simulink model "TesteEloGhendy"  (R2021b)
settings: Solver=FixedStepAuto  StartTime=0.0  StopTime=TempoSimulacao  RelTol=1e-3
values from neighbouring files (symbols this model uses):
  FatorSimulacao = 1e-3    (= 0.001)    [TesteRealCurtoFuses.m]    (also in TesteRealCurto_SemFuse.m)
  le = 1e-10    [TesteRealCurto.m]    (also in TesteRealCurtoFuses.m; TesteRealCurto_SemFuse.m)
  lm = (imag(Zm)/(2*pi*f))*d    [TesteRealCurto.m]    (also in TesteRealCurtoFuses.m; TesteRealCurto_SemFuse.m)
  lp = (imag(Zp)/(2*pi*f))*d    [TesteRealCurto.m]    (also in TesteRealCurtoFuses.m; TesteRealCurto_SemFuse.m)
  NRE = 1e-12    [TesteRealCurto.m]    (also in TesteRealCurtoFuses.m; TesteRealCurto_SemFuse.m)
  rm = real(Zm)*d    [TesteRealCurto.m]    (also in TesteRealCurtoFuses.m; TesteRealCurto_SemFuse.m)
  rp = real(Zp)*d    [TesteRealCurto.m]    (also in TesteRealCurtoFuses.m; TesteRealCurto_SemFuse.m)
  rtc = 10    [TesteRealCurto.m]    (also in TesteRealCurtoFuses.m; TesteRealCurto_SemFuse.m)
  rti = 10    [TesteRealCurto.m]    (also in TesteRealCurtoFuses.m; TesteRealCurto_SemFuse.m)
undefined symbols (not defined in the file or in its folder): D11, Delta, POT, PotConsumidor, Ra_Curto, Rb_Curto, Rc_Curto
libraries: spsRMSLib x15, spsBreakerLib x7, spsCurrentMeasurementLib x7, spsSeriesRLCBranchLib x6, spsThreePhaseVIMeasurementLib x4, spsThreePhaseTransformerTwoWindingsLib x2, spsThreePhaseSeriesRLCLoadLib x1, spsThreePhaseBreakerLib x1, spsThreePhaseSourceLib x1, spsMutualInductanceLib x1, spspowerguiLib x1
(part 2 of 2)

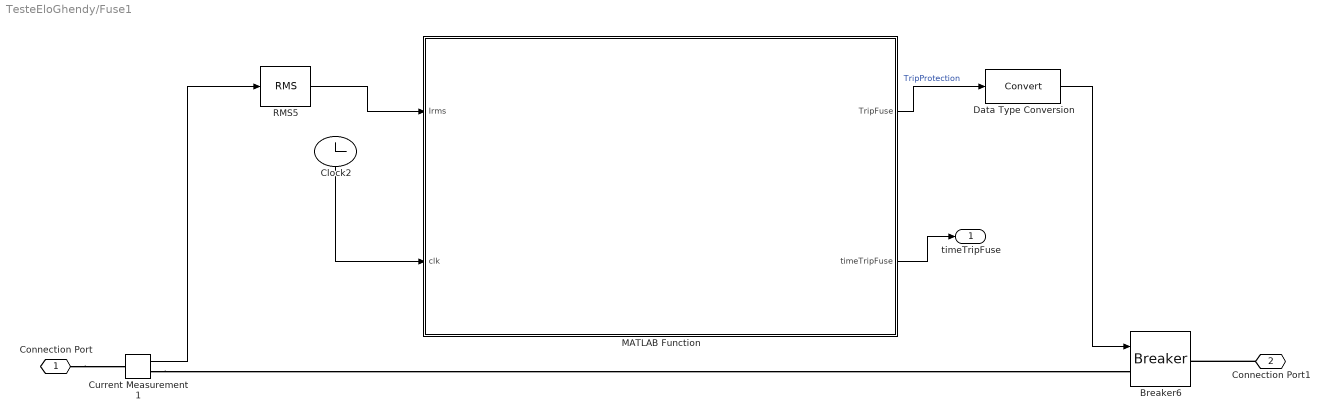
== system TesteEloGhendy/Fuse1 ==
  Breaker6 : spsBreakerLib/Breaker  InitialState=1  SwitchingTimes="[1/60  5/60]"  External=on  BreakerResistance=0.01  SnubberResistance=1e6  SnubberCapacitance=inf  Measurements=None  MoreParameters=on  NoBreakLoop=off
      settings: SourceProductBaseCode=PS
  Clock2 : Clock
      settings: Decimation=1000
  Current Measurement1 : spsCurrentMeasurementLib/Current Measurement  PhasorSimulation=off  OutputType=Complex  PSBequivalent=0
  Data Type Conversion : DataTypeConversion
  MATLAB Function : MATLAB Function
  RMS5 : spsRMSLib/RMS  TrueRMS=on  Freq=60  RMSInit=0  Ts=0
  Connection Port : PMIOPort  Side=Right
  Connection Port1 : PMIOPort  Port=2  Side=Left
  timeTripFuse : Outport
  wires:
  MATLAB Function/1(TripFuse) -> Data Type Conversion/1  "TripProtection"
  RMS5/1 -> MATLAB Function/1(Irms)
  Data Type Conversion/1 -> Breaker6/1
  Current Measurement1/1 -> RMS5/1
  Clock2/1 -> MATLAB Function/2(clk)
  MATLAB Function/2(timeTripFuse) -> timeTripFuse/1
  connections:
  Current Measurement1/RConn1 -- Breaker6/LConn1
  Connection Port/RConn1 -- Current Measurement1/LConn1
  Connection Port1/RConn1 -- Breaker6/RConn1

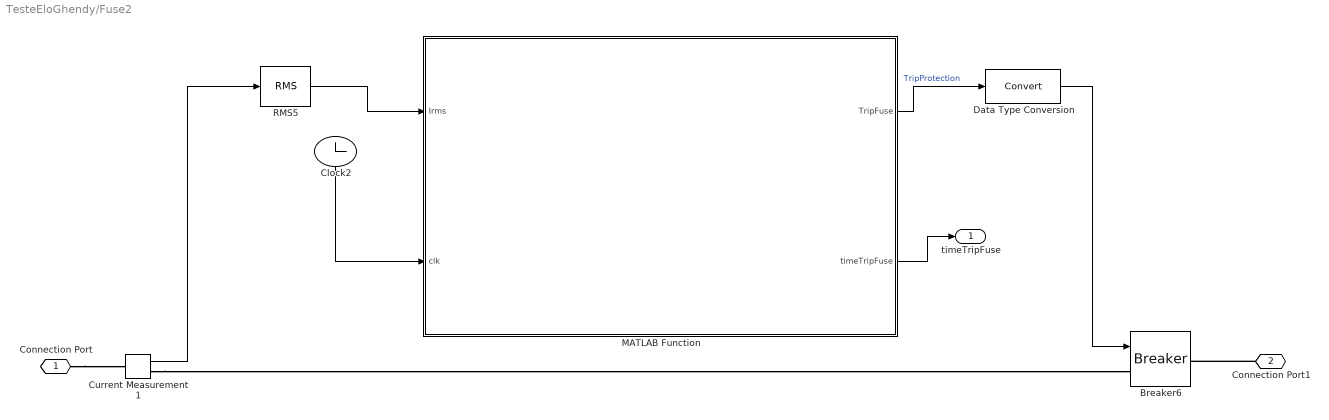
== system TesteEloGhendy/Fuse2 ==
  Breaker6 : spsBreakerLib/Breaker  InitialState=1  SwitchingTimes="[1/60  5/60]"  External=on  BreakerResistance=0.01  SnubberResistance=1e6  SnubberCapacitance=inf  Measurements=None  MoreParameters=on  NoBreakLoop=off
      settings: SourceProductBaseCode=PS
  Clock2 : Clock
      settings: Decimation=1000
  Current Measurement1 : spsCurrentMeasurementLib/Current Measurement  PhasorSimulation=off  OutputType=Complex  PSBequivalent=0
  Data Type Conversion : DataTypeConversion
  MATLAB Function : MATLAB Function
  RMS5 : spsRMSLib/RMS  TrueRMS=on  Freq=60  RMSInit=0  Ts=0
  Connection Port : PMIOPort  Side=Right
  Connection Port1 : PMIOPort  Port=2  Side=Left
  timeTripFuse : Outport
  wires:
  MATLAB Function/1(TripFuse) -> Data Type Conversion/1  "TripProtection"
  RMS5/1 -> MATLAB Function/1(Irms)
  Data Type Conversion/1 -> Breaker6/1
  Current Measurement1/1 -> RMS5/1
  Clock2/1 -> MATLAB Function/2(clk)
  MATLAB Function/2(timeTripFuse) -> timeTripFuse/1
  connections:
  Current Measurement1/RConn1 -- Breaker6/LConn1
  Connection Port/RConn1 -- Current Measurement1/LConn1
  Connection Port1/RConn1 -- Breaker6/RConn1

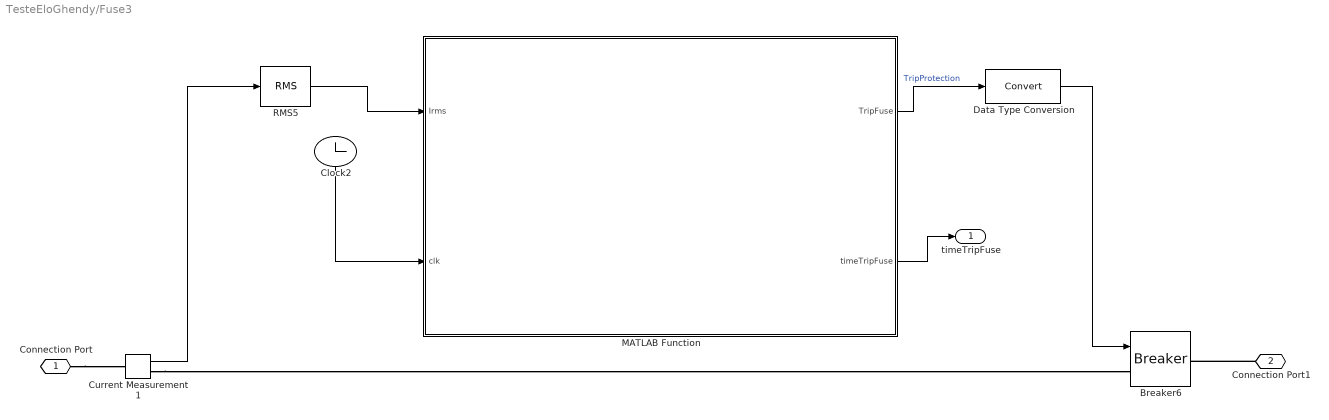
== system TesteEloGhendy/Fuse3 ==
  Breaker6 : spsBreakerLib/Breaker  InitialState=1  SwitchingTimes="[1/60  5/60]"  External=on  BreakerResistance=0.01  SnubberResistance=1e6  SnubberCapacitance=inf  Measurements=None  MoreParameters=on  NoBreakLoop=off
      settings: SourceProductBaseCode=PS
  Clock2 : Clock
      settings: Decimation=1000
  Current Measurement1 : spsCurrentMeasurementLib/Current Measurement  PhasorSimulation=off  OutputType=Complex  PSBequivalent=0
  Data Type Conversion : DataTypeConversion
  MATLAB Function : MATLAB Function
  RMS5 : spsRMSLib/RMS  TrueRMS=on  Freq=60  RMSInit=0  Ts=0
  Connection Port : PMIOPort  Side=Right
  Connection Port1 : PMIOPort  Port=2  Side=Left
  timeTripFuse : Outport
  wires:
  MATLAB Function/1(TripFuse) -> Data Type Conversion/1  "TripProtection"
  RMS5/1 -> MATLAB Function/1(Irms)
  Data Type Conversion/1 -> Breaker6/1
  Current Measurement1/1 -> RMS5/1
  Clock2/1 -> MATLAB Function/2(clk)
  MATLAB Function/2(timeTripFuse) -> timeTripFuse/1
  connections:
  Current Measurement1/RConn1 -- Breaker6/LConn1
  Connection Port/RConn1 -- Current Measurement1/LConn1
  Connection Port1/RConn1 -- Breaker6/RConn1

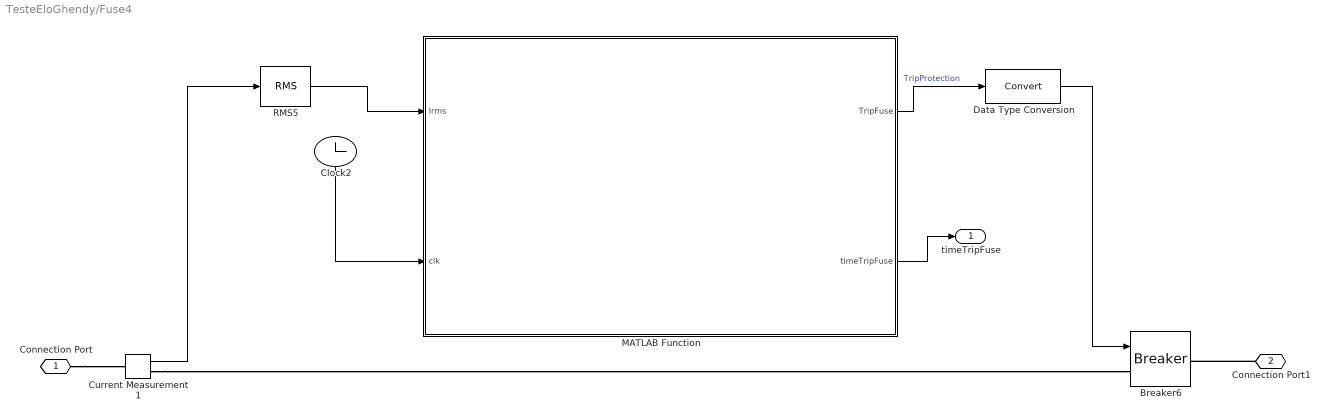
== system TesteEloGhendy/Fuse4 ==
  Breaker6 : spsBreakerLib/Breaker  InitialState=1  SwitchingTimes="[1/60  5/60]"  External=on  BreakerResistance=0.01  SnubberResistance=1e6  SnubberCapacitance=inf  Measurements=None  MoreParameters=on  NoBreakLoop=off
      settings: SourceProductBaseCode=PS
  Clock2 : Clock
      settings: Decimation=1000
  Current Measurement1 : spsCurrentMeasurementLib/Current Measurement  PhasorSimulation=off  OutputType=Complex  PSBequivalent=0
  Data Type Conversion : DataTypeConversion
  MATLAB Function : MATLAB Function
  RMS5 : spsRMSLib/RMS  TrueRMS=on  Freq=60  RMSInit=0  Ts=0
  Connection Port : PMIOPort  Side=Right
  Connection Port1 : PMIOPort  Port=2  Side=Left
  timeTripFuse : Outport
  wires:
  MATLAB Function/1(TripFuse) -> Data Type Conversion/1  "TripProtection"
  RMS5/1 -> MATLAB Function/1(Irms)
  Data Type Conversion/1 -> Breaker6/1
  Current Measurement1/1 -> RMS5/1
  Clock2/1 -> MATLAB Function/2(clk)
  MATLAB Function/2(timeTripFuse) -> timeTripFuse/1
  connections:
  Current Measurement1/RConn1 -- Breaker6/LConn1
  Connection Port/RConn1 -- Current Measurement1/LConn1
  Connection Port1/RConn1 -- Breaker6/RConn1

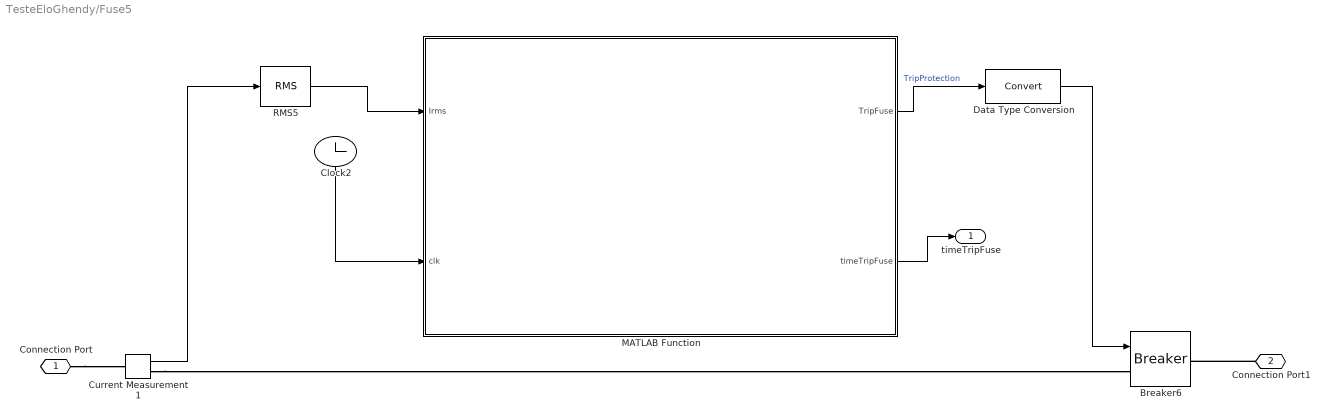
== system TesteEloGhendy/Fuse5 ==
  Breaker6 : spsBreakerLib/Breaker  InitialState=1  SwitchingTimes="[1/60  5/60]"  External=on  BreakerResistance=0.01  SnubberResistance=1e6  SnubberCapacitance=inf  Measurements=None  MoreParameters=on  NoBreakLoop=off
      settings: SourceProductBaseCode=PS
  Clock2 : Clock
      settings: Decimation=1000
  Current Measurement1 : spsCurrentMeasurementLib/Current Measurement  PhasorSimulation=off  OutputType=Complex  PSBequivalent=0
  Data Type Conversion : DataTypeConversion
  MATLAB Function : MATLAB Function
  RMS5 : spsRMSLib/RMS  TrueRMS=on  Freq=60  RMSInit=0  Ts=0
  Connection Port : PMIOPort  Side=Right
  Connection Port1 : PMIOPort  Port=2  Side=Left
  timeTripFuse : Outport
  wires:
  MATLAB Function/1(TripFuse) -> Data Type Conversion/1  "TripProtection"
  RMS5/1 -> MATLAB Function/1(Irms)
  Data Type Conversion/1 -> Breaker6/1
  Current Measurement1/1 -> RMS5/1
  Clock2/1 -> MATLAB Function/2(clk)
  MATLAB Function/2(timeTripFuse) -> timeTripFuse/1
  connections:
  Current Measurement1/RConn1 -- Breaker6/LConn1
  Connection Port/RConn1 -- Current Measurement1/LConn1
  Connection Port1/RConn1 -- Breaker6/RConn1

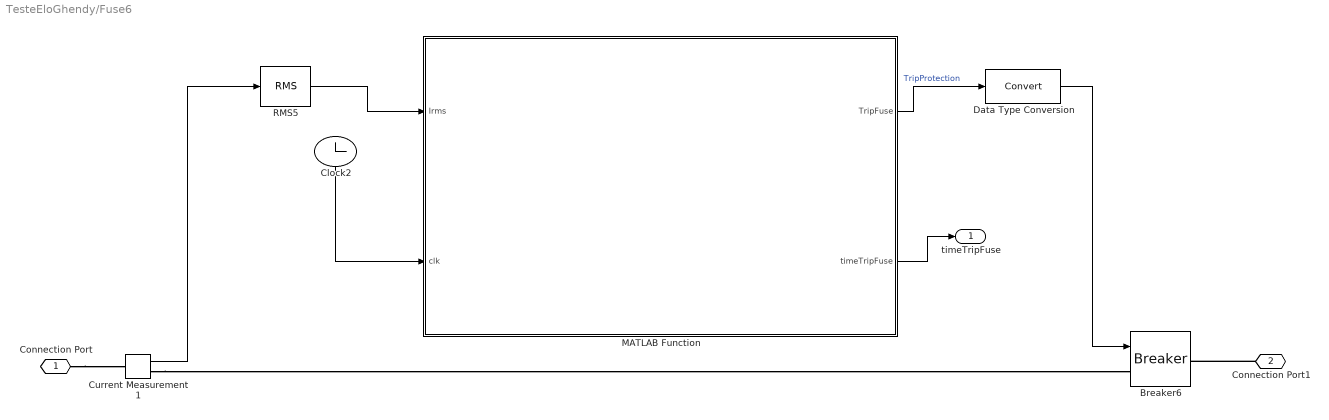
== system TesteEloGhendy/Fuse6 ==
  Breaker6 : spsBreakerLib/Breaker  InitialState=1  SwitchingTimes="[1/60  5/60]"  External=on  BreakerResistance=0.01  SnubberResistance=1e6  SnubberCapacitance=inf  Measurements=None  MoreParameters=on  NoBreakLoop=off
      settings: SourceProductBaseCode=PS
  Clock2 : Clock
      settings: Decimation=1000
  Current Measurement1 : spsCurrentMeasurementLib/Current Measurement  PhasorSimulation=off  OutputType=Complex  PSBequivalent=0
  Data Type Conversion : DataTypeConversion
  MATLAB Function : MATLAB Function
  RMS5 : spsRMSLib/RMS  TrueRMS=on  Freq=60  RMSInit=0  Ts=0
  Connection Port : PMIOPort  Side=Right
  Connection Port1 : PMIOPort  Port=2  Side=Left
  timeTripFuse : Outport
  wires:
  MATLAB Function/1(TripFuse) -> Data Type Conversion/1  "TripProtection"
  RMS5/1 -> MATLAB Function/1(Irms)
  Data Type Conversion/1 -> Breaker6/1
  Current Measurement1/1 -> RMS5/1
  Clock2/1 -> MATLAB Function/2(clk)
  MATLAB Function/2(timeTripFuse) -> timeTripFuse/1
  connections:
  Current Measurement1/RConn1 -- Breaker6/LConn1
  Connection Port/RConn1 -- Current Measurement1/LConn1
  Connection Port1/RConn1 -- Breaker6/RConn1

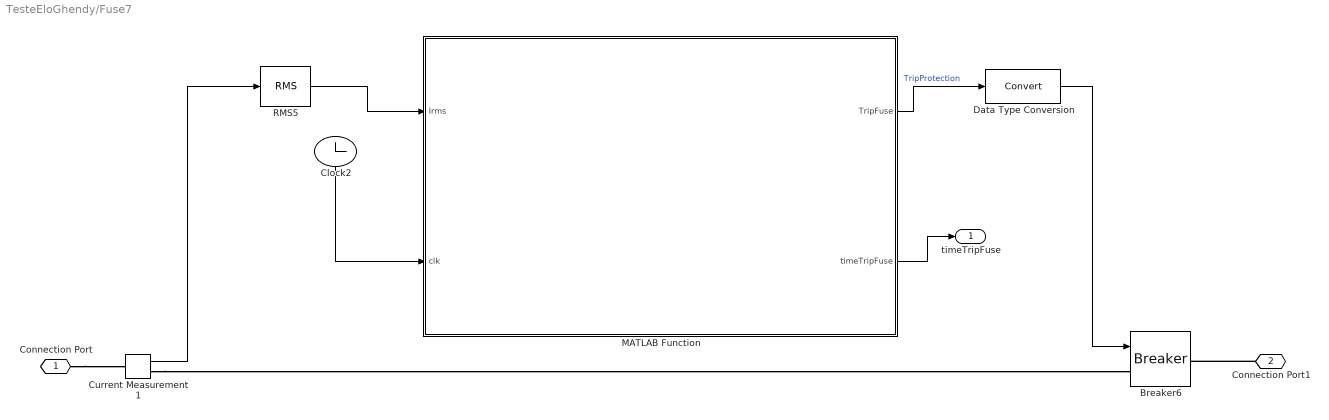
== system TesteEloGhendy/Fuse7 ==
  Breaker6 : spsBreakerLib/Breaker  InitialState=1  SwitchingTimes="[1/60  5/60]"  External=on  BreakerResistance=0.01  SnubberResistance=1e6  SnubberCapacitance=inf  Measurements=None  MoreParameters=on  NoBreakLoop=off
      settings: SourceProductBaseCode=PS
  Clock2 : Clock
      settings: Decimation=1000
  Current Measurement1 : spsCurrentMeasurementLib/Current Measurement  PhasorSimulation=off  OutputType=Complex  PSBequivalent=0
  Data Type Conversion : DataTypeConversion
  MATLAB Function : MATLAB Function
  RMS5 : spsRMSLib/RMS  TrueRMS=on  Freq=60  RMSInit=0  Ts=0
  Connection Port : PMIOPort  Side=Right
  Connection Port1 : PMIOPort  Port=2  Side=Left
  timeTripFuse : Outport
  wires:
  MATLAB Function/1(TripFuse) -> Data Type Conversion/1  "TripProtection"
  RMS5/1 -> MATLAB Function/1(Irms)
  Data Type Conversion/1 -> Breaker6/1
  Current Measurement1/1 -> RMS5/1
  Clock2/1 -> MATLAB Function/2(clk)
  MATLAB Function/2(timeTripFuse) -> timeTripFuse/1
  connections:
  Current Measurement1/RConn1 -- Breaker6/LConn1
  Connection Port/RConn1 -- Current Measurement1/LConn1
  Connection Port1/RConn1 -- Breaker6/RConn1

== matlab function TesteEloGhendy/Fuse6/MATLAB Function ==
  settings: updateMethod=DISCRETE
  data: Irms input; clk input; TripFuse output; a parameter; b parameter; c parameter; d parameter; e parameter; timeTripFuse output; IoTot parameter
function [TripFuse, timeTripFuse ]  =  fcn(Irms, clk, a, b, c, d, e, IoTot)
persistent RelayStateOvercurrentTime OperatingTime PickupTime TripTime signal valorIRMS y t timeTrip ValorAbertura
if isempty(RelayStateOvercurrentTime)
    RelayStateOvercurrentTime = 0;
    TripTime = 0;
    signal = 1;
    OperatingTime = inf;
    PickupTime = 0;
    valorIRMS = 0;
    timeTrip = inf;
    ValorAbertura = inf;
end

%% tripFuse
if (RelayStateOvercurrentTime == 0)&&(Irms > IoTot*3)
    PickupTime = clk+0.07;
    RelayStateOvercurrentTime = 1;
end

if(RelayStateOvercurrentTime == 1)&&(clk>PickupTime)
    valorIRMS = Irms;
    y = log(valorIRMS);
    t = a + (b * y) + (c * y^2) + (d * y^3) + (e * y^4);
    OperatingTime = exp(t);
    TripTime = PickupTime + OperatingTime;
    RelayStateOvercurrentTime = 2;
end

if (clk > TripTime)&&(RelayStateOvercurrentTime == 2)
    if ((Irms <= valorIRMS*0.5)&&(Irms <= IoTot*3))
        signal = 1;
        RelayStateOvercurrentTime = 0;
        TripTime = inf;
    else
        ValorAbertura = clk;
        signal = 0;
        RelayStateOvercurrentTime = 3;
        timeTrip = OperatingTime;
    end
end

TripFuse = signal;
timeTripFuse = [valorIRMS timeTrip ValorAbertura];

== matlab function TesteEloGhendy/Fuse7/MATLAB Function ==
  settings: updateMethod=DISCRETE
  data: Irms input; clk input; TripFuse output; a parameter; b parameter; c parameter; d parameter; e parameter; timeTripFuse output; IoTot parameter
function [TripFuse, timeTripFuse ]  =  fcn(Irms, clk, a, b, c, d, e, IoTot)
persistent RelayStateOvercurrentTime OperatingTime PickupTime TripTime signal valorIRMS y t timeTrip ValorAbertura
if isempty(RelayStateOvercurrentTime)
    RelayStateOvercurrentTime = 0;
    TripTime = 0;
    signal = 1;
    OperatingTime = inf;
    PickupTime = 0;
    valorIRMS = 0;
    timeTrip = inf;
    ValorAbertura = inf;
end

%% tripFuse
if (RelayStateOvercurrentTime == 0)&&(Irms > IoTot*3)
    PickupTime = clk+0.07;
    RelayStateOvercurrentTime = 1;
end

if(RelayStateOvercurrentTime == 1)&&(clk>PickupTime)
    valorIRMS = Irms;
    y = log(valorIRMS);
    t = a + (b * y) + (c * y^2) + (d * y^3) + (e * y^4);
    OperatingTime = exp(t);
    TripTime = PickupTime + OperatingTime;
    RelayStateOvercurrentTime = 2;
end

if (clk > TripTime)&&(RelayStateOvercurrentTime == 2)
    if ((Irms <= valorIRMS*0.5)&&(Irms <= IoTot*3))
        signal = 1;
        RelayStateOvercurrentTime = 0;
        TripTime = inf;
    else
        ValorAbertura = clk;
        signal = 0;
        RelayStateOvercurrentTime = 3;
        timeTrip = OperatingTime;
    end
end

TripFuse = signal;
timeTripFuse = [valorIRMS timeTrip ValorAbertura];

== matlab function TesteEloGhendy/Fuse1/MATLAB Function ==
  settings: updateMethod=DISCRETE
  data: Irms input; clk input; TripFuse output; a parameter; b parameter; c parameter; d parameter; e parameter; timeTripFuse output; IoTot parameter
function [TripFuse, timeTripFuse ]  =  fcn(Irms, clk, a, b, c, d, e, IoTot)
persistent RelayStateOvercurrentTime OperatingTime PickupTime TripTime signal valorIRMS y t timeTrip ValorAbertura
if isempty(RelayStateOvercurrentTime)
    RelayStateOvercurrentTime = 0;
    TripTime = 0;
    signal = 1;
    OperatingTime = inf;
    PickupTime = 0;
    valorIRMS = 0;
    timeTrip = inf;
    ValorAbertura = inf;
end

%% tripFuse
if (RelayStateOvercurrentTime == 0)&&(Irms > IoTot*3)
    PickupTime = clk+0.07;
    RelayStateOvercurrentTime = 1;
end

if(RelayStateOvercurrentTime == 1)&&(clk>PickupTime)
    valorIRMS = Irms;
    y = log(valorIRMS);
    t = a + (b * y) + (c * y^2) + (d * y^3) + (e * y^4);
    OperatingTime = exp(t);
    TripTime = PickupTime + OperatingTime;
    RelayStateOvercurrentTime = 2;
end

if (clk > TripTime)&&(RelayStateOvercurrentTime == 2)
    if ((Irms <= valorIRMS*0.5)&&(Irms <= IoTot*3))
        signal = 1;
        RelayStateOvercurrentTime = 0;
        TripTime = inf;
    else
        ValorAbertura = clk;
        signal = 0;
        RelayStateOvercurrentTime = 3;
        timeTrip = OperatingTime;
    end
end

TripFuse = signal;
timeTripFuse = [valorIRMS timeTrip ValorAbertura];

== matlab function TesteEloGhendy/Fuse2/MATLAB Function ==
  settings: updateMethod=DISCRETE
  data: Irms input; clk input; TripFuse output; a parameter; b parameter; c parameter; d parameter; e parameter; timeTripFuse output; IoTot parameter
function [TripFuse, timeTripFuse ]  =  fcn(Irms, clk, a, b, c, d, e, IoTot)
persistent RelayStateOvercurrentTime OperatingTime PickupTime TripTime signal valorIRMS y t timeTrip ValorAbertura
if isempty(RelayStateOvercurrentTime)
    RelayStateOvercurrentTime = 0;
    TripTime = 0;
    signal = 1;
    OperatingTime = inf;
    PickupTime = 0;
    valorIRMS = 0;
    timeTrip = inf;
    ValorAbertura = inf;
end

%% tripFuse
if (RelayStateOvercurrentTime == 0)&&(Irms > IoTot*3)
    PickupTime = clk+0.07;
    RelayStateOvercurrentTime = 1;
end

if(RelayStateOvercurrentTime == 1)&&(clk>PickupTime)
    valorIRMS = Irms;
    y = log(valorIRMS);
    t = a + (b * y) + (c * y^2) + (d * y^3) + (e * y^4);
    OperatingTime = exp(t);
    TripTime = PickupTime + OperatingTime;
    RelayStateOvercurrentTime = 2;
end

if (clk > TripTime)&&(RelayStateOvercurrentTime == 2)
    if ((Irms <= valorIRMS*0.5)&&(Irms <= IoTot*3))
        signal = 1;
        RelayStateOvercurrentTime = 0;
        TripTime = inf;
    else
        ValorAbertura = clk;
        signal = 0;
        RelayStateOvercurrentTime = 3;
        timeTrip = OperatingTime;
    end
end

TripFuse = signal;
timeTripFuse = [valorIRMS timeTrip ValorAbertura];

== matlab function TesteEloGhendy/Fuse3/MATLAB Function ==
  settings: updateMethod=DISCRETE
  data: Irms input; clk input; TripFuse output; a parameter; b parameter; c parameter; d parameter; e parameter; timeTripFuse output; IoTot parameter
function [TripFuse, timeTripFuse ]  =  fcn(Irms, clk, a, b, c, d, e, IoTot)
persistent RelayStateOvercurrentTime OperatingTime PickupTime TripTime signal valorIRMS y t timeTrip ValorAbertura
if isempty(RelayStateOvercurrentTime)
    RelayStateOvercurrentTime = 0;
    TripTime = 0;
    signal = 1;
    OperatingTime = inf;
    PickupTime = 0;
    valorIRMS = 0;
    timeTrip = inf;
    ValorAbertura = inf;
end

%% tripFuse
if (RelayStateOvercurrentTime == 0)&&(Irms > IoTot*3)
    PickupTime = clk+0.07;
    RelayStateOvercurrentTime = 1;
end

if(RelayStateOvercurrentTime == 1)&&(clk>PickupTime)
    valorIRMS = Irms;
    y = log(valorIRMS);
    t = a + (b * y) + (c * y^2) + (d * y^3) + (e * y^4);
    OperatingTime = exp(t);
    TripTime = PickupTime + OperatingTime;
    RelayStateOvercurrentTime = 2;
end

if (clk > TripTime)&&(RelayStateOvercurrentTime == 2)
    if ((Irms <= valorIRMS*0.5)&&(Irms <= IoTot*3))
        signal = 1;
        RelayStateOvercurrentTime = 0;
        TripTime = inf;
    else
        ValorAbertura = clk;
        signal = 0;
        RelayStateOvercurrentTime = 3;
        timeTrip = OperatingTime;
    end
end

TripFuse = signal;
timeTripFuse = [valorIRMS timeTrip ValorAbertura];

== matlab function TesteEloGhendy/Fuse4/MATLAB Function ==
  settings: updateMethod=DISCRETE
  data: Irms input; clk input; TripFuse output; a parameter; b parameter; c parameter; d parameter; e parameter; timeTripFuse output; IoTot parameter
function [TripFuse, timeTripFuse ]  =  fcn(Irms, clk, a, b, c, d, e, IoTot)
persistent RelayStateOvercurrentTime OperatingTime PickupTime TripTime signal valorIRMS y t timeTrip ValorAbertura
if isempty(RelayStateOvercurrentTime)
    RelayStateOvercurrentTime = 0;
    TripTime = 0;
    signal = 1;
    OperatingTime = inf;
    PickupTime = 0;
    valorIRMS = 0;
    timeTrip = inf;
    ValorAbertura = inf;
end

%% tripFuse
if (RelayStateOvercurrentTime == 0)&&(Irms > IoTot*3)
    PickupTime = clk+0.07;
    RelayStateOvercurrentTime = 1;
end

if(RelayStateOvercurrentTime == 1)&&(clk>PickupTime)
    valorIRMS = Irms;
    y = log(valorIRMS);
    t = a + (b * y) + (c * y^2) + (d * y^3) + (e * y^4);
    OperatingTime = exp(t);
    TripTime = PickupTime + OperatingTime;
    RelayStateOvercurrentTime = 2;
end

if (clk > TripTime)&&(RelayStateOvercurrentTime == 2)
    if ((Irms <= valorIRMS*0.5)&&(Irms <= IoTot*3))
        signal = 1;
        RelayStateOvercurrentTime = 0;
        TripTime = inf;
    else
        ValorAbertura = clk;
        signal = 0;
        RelayStateOvercurrentTime = 3;
        timeTrip = OperatingTime;
    end
end

TripFuse = signal;
timeTripFuse = [valorIRMS timeTrip ValorAbertura];

== matlab function TesteEloGhendy/Fuse5/MATLAB Function ==
  settings: updateMethod=DISCRETE
  data: Irms input; clk input; TripFuse output; a parameter; b parameter; c parameter; d parameter; e parameter; timeTripFuse output; IoTot parameter
function [TripFuse, timeTripFuse ]  =  fcn(Irms, clk, a, b, c, d, e, IoTot)
persistent RelayStateOvercurrentTime OperatingTime PickupTime TripTime signal valorIRMS y t timeTrip ValorAbertura
if isempty(RelayStateOvercurrentTime)
    RelayStateOvercurrentTime = 0;
    TripTime = 0;
    signal = 1;
    OperatingTime = inf;
    PickupTime = 0;
    valorIRMS = 0;
    timeTrip = inf;
    ValorAbertura = inf;
end

%% tripFuse
if (RelayStateOvercurrentTime == 0)&&(Irms > IoTot*3)
    PickupTime = clk+0.07;
    RelayStateOvercurrentTime = 1;
end

if(RelayStateOvercurrentTime == 1)&&(clk>PickupTime)
    valorIRMS = Irms;
    y = log(valorIRMS);
    t = a + (b * y) + (c * y^2) + (d * y^3) + (e * y^4);
    OperatingTime = exp(t);
    TripTime = PickupTime + OperatingTime;
    RelayStateOvercurrentTime = 2;
end

if (clk > TripTime)&&(RelayStateOvercurrentTime == 2)
    if ((Irms <= valorIRMS*0.5)&&(Irms <= IoTot*3))
        signal = 1;
        RelayStateOvercurrentTime = 0;
        TripTime = inf;
    else
        ValorAbertura = clk;
        signal = 0;
        RelayStateOvercurrentTime = 3;
        timeTrip = OperatingTime;
    end
end

TripFuse = signal;
timeTripFuse = [valorIRMS timeTrip ValorAbertura];
